simulink library "ITKLib"  (R2022b)
settings: Solver=FixedStepDiscrete  StartTime=0.0  StopTime=10.0  FixedStep=0.01  RelTol=1e-3  EnableMultiTasking=on
values from neighbouring files (symbols this model uses):
  Glb_WhlRollgRd_SC = single(0.36)    [init_Global.m]
undefined symbols (not defined in the file or in its folder): docblock, SlDemoSign, SlDemoSign_Positive_SC, TaskTime_100ms_SC, TaskTime_10ms_SC, VehRefSpd_vMaxRefSpd_C
libraries: simulink x51, $bdroot x45, ITKLib_V14 x1
(part 5 of 10)

== system ITKLib/BasicOperators/SinDeg ==
  deg : Inport
  1-D Lookup Table1 : Lookup_n-D  NumberOfTableDimensions=1  BreakpointsForDimension1=[0,5,10,15,20,25,30,35,40,45,50,55,60,65,70,75,80,85,90]  BreakpointsForDimension1DataTypeStr=single  Table=[0,0.0871557427476582,0.173648177666930,0.258819045102521,0.342020143325669,0.422618261740699,0.500000000000000,0.573576436351046,0.642787609686539,0.707106781186548,0.766044443118978,0.819152044288992,0.866025403784439,0.906307787036650,0.939692620785908,0.965925826289068,0.984807753012208,0.996194698091746,1]  TableDataTypeStr=single  IntermediateResultsDataTypeStr=single  ExtrapMethod=Clip  UseLastTableValue=on  InternalRulePriority=Speed  OutDataTypeStr=single  RndMeth=Simplest  FractionDataTypeStr=single
      settings: AttributesFormatString=|
      | input = %<BreakpointsForDimension1>
      | output = %<Table>
      | extrapolation-use end values: %<UseLastTableValue>
  1-D Lookup Table2 : Lookup_n-D  NumberOfTableDimensions=1  BreakpointsForDimension1=[0,5,10,15,20,25,30,35,40,45,50,55,60,65,70,75,80,85,90]  BreakpointsForDimension1DataTypeStr=single  Table=[0,0.0871557427476582,0.173648177666930,0.258819045102521,0.342020143325669,0.422618261740699,0.500000000000000,0.573576436351046,0.642787609686539,0.707106781186548,0.766044443118978,0.819152044288992,0.866025403784439,0.906307787036650,0.939692620785908,0.965925826289068,0.984807753012208,0.996194698091746,1]  TableDataTypeStr=single  IntermediateResultsDataTypeStr=single  ExtrapMethod=Clip  UseLastTableValue=on  InternalRulePriority=Speed  OutDataTypeStr=single  RndMeth=Simplest  FractionDataTypeStr=single
      settings: AttributesFormatString=|
      | input = %<BreakpointsForDimension1>
      | output = %<Table>
      | extrapolation-use end values: %<UseLastTableValue>
  AbsITK : $bdroot/BasicOperators/AbsITK
  AbsITK1 : $bdroot/BasicOperators/AbsITK
  Divide : Product  Inputs=*/  InputSameDT=on  RndMeth=Zero  SaturateOnIntegerOverflow=on
  GreaterOrEqual{,1..3} (4 alike) : RelationalOperator  OutDataTypeStr=boolean
  GreaterOrEqual4 : RelationalOperator  Operator=<=  OutDataTypeStr=boolean
  GreaterOrEqual5 : RelationalOperator  Operator=<=  OutDataTypeStr=boolean
  GreaterOrEqual6 : RelationalOperator  Operator=<=  OutDataTypeStr=boolean
  Multiport Switch{1..4} (4 alike) : MultiPortSwitch  Inputs=4  SaturateOnIntegerOverflow=off  InputSameDT=off
  Product : Product  InputSameDT=on  RndMeth=Zero  SaturateOnIntegerOverflow=on
  Product1 : Product  InputSameDT=on  RndMeth=Zero  SaturateOnIntegerOverflow=on
  Product2 : Product  InputSameDT=on  RndMeth=Zero  SaturateOnIntegerOverflow=on
  Rounding Function : Rounding  Operator=fix
  Subtract{,1..3} (4 alike) : Sum  Inputs=+-  InputSameDT=on  SaturateOnIntegerOverflow=on
  Subtract4 : Sum  InputSameDT=on  SaturateOnIntegerOverflow=on
  Subtract5 : Sum  InputSameDT=on  SaturateOnIntegerOverflow=on
  Switch{1..7} (7 alike) : Switch  Criteria=u2 ~= 0  SaturateOnIntegerOverflow=off  InputSameDT=off
      settings: AttributesFormatString=Criteria : %<Criteria>
  single1 : Constant  Value=360  OutDataTypeStr=single
      settings: AttributesFormatString=%<OutDataTypeStr>
  single{6,10,14,17} (4 alike) : Constant  Value=180  OutDataTypeStr=single
      settings: AttributesFormatString=%<OutDataTypeStr>
  single11 : Constant  Value=90  OutDataTypeStr=single
      settings: AttributesFormatString=%<OutDataTypeStr>
  single12 : Constant  Value=270  OutDataTypeStr=single
      settings: AttributesFormatString=%<OutDataTypeStr>
  single15 : Constant  Value=360  OutDataTypeStr=single
      settings: AttributesFormatString=%<OutDataTypeStr>
  single19 : Constant  Value=360  OutDataTypeStr=single
      settings: AttributesFormatString=%<OutDataTypeStr>
  single2 : Constant  Value=0  OutDataTypeStr=single
      settings: AttributesFormatString=%<OutDataTypeStr>
  single20 : Constant  OutDataTypeStr=single
      settings: AttributesFormatString=%<OutDataTypeStr>
  single21 : Constant  Value=-1  OutDataTypeStr=single
      settings: AttributesFormatString=%<OutDataTypeStr>
  single3 : Constant  Value=-180  OutDataTypeStr=single
      settings: AttributesFormatString=%<OutDataTypeStr>
  single4 : Constant  Value=-90  OutDataTypeStr=single
      settings: AttributesFormatString=%<OutDataTypeStr>
  single5 : Constant  Value=-270  OutDataTypeStr=single
      settings: AttributesFormatString=%<OutDataTypeStr>
  single7 : Constant  OutDataTypeStr=single
      settings: AttributesFormatString=%<OutDataTypeStr>
  single8 : Constant  Value=-1  OutDataTypeStr=single
      settings: AttributesFormatString=%<OutDataTypeStr>
  uint1 : Constant  OutDataTypeStr=uint8
      settings: AttributesFormatString=%<OutDataTypeStr>
  uint2 : Constant  Value=4  OutDataTypeStr=uint8
      settings: AttributesFormatString=%<OutDataTypeStr>
  uint3 : Constant  Value=3  OutDataTypeStr=uint8
      settings: AttributesFormatString=%<OutDataTypeStr>
  uint4 : Constant  Value=2  OutDataTypeStr=uint8
      settings: AttributesFormatString=%<OutDataTypeStr>
  uint5 : Constant  OutDataTypeStr=uint8
      settings: AttributesFormatString=%<OutDataTypeStr>
  uint6 : Constant  Value=2  OutDataTypeStr=uint8
      settings: AttributesFormatString=%<OutDataTypeStr>
  uint7 : Constant  Value=3  OutDataTypeStr=uint8
      settings: AttributesFormatString=%<OutDataTypeStr>
  uint8 : Constant  Value=4  OutDataTypeStr=uint8
      settings: AttributesFormatString=%<OutDataTypeStr>
  out : Outport
  wires:
  Subtract2/1 -> Multiport Switch1/5
  single15/1 -> Subtract2/1
  Subtract1/1 -> Multiport Switch1/4
  single14/1 -> Subtract1/2
  single8/1 -> Multiport Switch2/4, Multiport Switch2/5
  single7/1 -> Multiport Switch2/2, Multiport Switch2/3
  Product1/1 -> Switch1/1
  Multiport Switch2/1 -> Product1/1
  single6/1 -> Subtract/1
  Subtract/1 -> Multiport Switch1/3
  Multiport Switch1/1 -> 1-D Lookup Table2/1
  uint5/1 -> Switch4/3
  uint4/1 -> Switch4/1
  Switch4/1 -> Switch3/3
  GreaterOrEqual2/1 -> Switch4/2
  single11/1 -> GreaterOrEqual2/2
  uint3/1 -> Switch3/1
  GreaterOrEqual1/1 -> Switch3/2
  single10/1 -> GreaterOrEqual1/2
  single12/1 -> GreaterOrEqual/2
  1-D Lookup Table2/1 -> Product1/2
  Switch2/1 -> Multiport Switch2/1, Multiport Switch1/1
  Switch3/1 -> Switch2/3
  uint2/1 -> Switch2/1
  GreaterOrEqual/1 -> Switch2/2
  Rounding Function/1 -> Product/1
  Product/1 -> Subtract3/2
  Divide/1 -> Rounding Function/1
  deg/1 -> Divide/1, Subtract3/1
  single1/1 -> Product/2, Divide/2
  single2/1 -> GreaterOrEqual3/2
  GreaterOrEqual3/1 -> Switch1/2
  Switch1/1 -> out/1
  GreaterOrEqual4/1 -> Switch5/2
  uint1/1 -> Switch5/1
  Switch6/1 -> Switch5/3
  Switch5/1 -> Multiport Switch4/1, Multiport Switch3/1
  1-D Lookup Table1/1 -> Product2/2
  single5/1 -> GreaterOrEqual4/2
  single3/1 -> GreaterOrEqual5/2
  GreaterOrEqual5/1 -> Switch6/2
  uint6/1 -> Switch6/1
  single4/1 -> GreaterOrEqual6/2
  GreaterOrEqual6/1 -> Switch7/2
  Switch7/1 -> Switch6/3
  uint7/1 -> Switch7/1
  uint8/1 -> Switch7/3
  Multiport Switch3/1 -> 1-D Lookup Table1/1
  Subtract4/1 -> Multiport Switch3/2
  Multiport Switch4/1 -> Product2/1
  Product2/1 -> Switch1/3
  single20/1 -> Multiport Switch4/3, Multiport Switch4/2
  single21/1 -> Multiport Switch4/5, Multiport Switch4/4
  Subtract3/1 -> GreaterOrEqual3/1, AbsITK1/1, Subtract5/1, Subtract4/1, GreaterOrEqual6/1, GreaterOrEqual5/1, GreaterOrEqual4/1, Subtract2/2, Subtract1/1, Subtract/2, Multiport Switch1/2, GreaterOrEqual2/1, GreaterOrEqual1/1, GreaterOrEqual/1
  single19/1 -> Subtract4/2
  single17/1 -> Subtract5/2
  Subtract5/1 -> AbsITK/1, Multiport Switch3/4
  AbsITK/1 -> Multiport Switch3/3
  AbsITK1/1 -> Multiport Switch3/5

== system ITKLib/BasicOperators/SingleToInt ==
  In : Inport  OutDataTypeStr=single
  FL : Inport  Port=2  OutDataTypeStr=single
  DataTypeConversion1 : DataTypeConversion  OutDataTypeStr=int32  RndMeth=Nearest
  Pow1 : Math  Operator=pow  SignedPower=on  RndMeth=Zero
  Product : Product  InputSameDT=on  SaturateOnIntegerOverflow=on
  single1 : Constant  Value=2  OutDataTypeStr=single  SampleTime=-1
      settings: AttributesFormatString=%<OutDataTypeStr>
  Out : Outport  OutDataTypeStr=int32
  wires:
  Product/1 -> DataTypeConversion1/1
  Pow1/1 -> Product/2
  single1/1 -> Pow1/1
  DataTypeConversion1/1 -> Out/1
  In/1 -> Product/1
  FL/1 -> Pow1/2

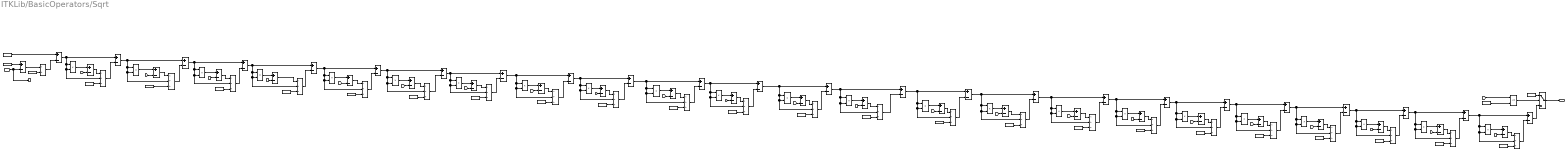
== system ITKLib/BasicOperators/Sqrt ==
  note: 牛顿法的迭代过程：
      | 对于任意方程F(X) = 0, 牛顿法的迭代过程可以描述为
      | Xn+1 = Xn - F(Xn) / F'(Xn)
  In : Inport
  Divide : Product  Inputs=*/  InputSameDT=on  SaturateOnIntegerOverflow=on
  Divide{1..23} (23 alike) : Product  Inputs=*//  InputSameDT=on  SaturateOnIntegerOverflow=on
  GreaterOrEqual : RelationalOperator  Operator=<=  OutDataTypeStr=boolean
  Product{,1..22} (23 alike) : Product  InputSameDT=on  SaturateOnIntegerOverflow=on
  Subtract{,1..47} (48 alike) : Sum  Inputs=+-  InputSameDT=on  SaturateOnIntegerOverflow=on
  Switch : Switch  Criteria=u2 ~= 0  SaturateOnIntegerOverflow=off  InputSameDT=off
      settings: AttributesFormatString=Criteria : %<Criteria>
  single : Constant  Value=0  OutDataTypeStr=single
      settings: AttributesFormatString=%<OutDataTypeStr>
  single1 : Constant  Value=0  OutDataTypeStr=single
      settings: AttributesFormatString=%<OutDataTypeStr>
  single{2,5..27} (24 alike) : Constant  Value=2  OutDataTypeStr=single
      settings: AttributesFormatString=%<OutDataTypeStr>
  single3 : Constant  Value=4  OutDataTypeStr=single
      settings: AttributesFormatString=%<OutDataTypeStr>
  single4 : Constant  Value=4  OutDataTypeStr=single
      settings: AttributesFormatString=%<OutDataTypeStr>
  Sqrt : Outport
  wires:
  single21/1 -> Divide17/3
  Product15/1 -> Subtract33/1
  Subtract36/1 -> Divide17/1
  [In] -> Subtract36/2
  Subtract22/1 -> Subtract24/1, Product11/1, Product11/2, Divide12/2
  Subtract32/1 -> Divide17/2, Product16/2, Product16/1, Subtract35/1
  Subtract28/1 -> Subtract30/1, Divide15/2, Product14/2, Product14/1
  single13/1 -> Divide9/3
  Subtract6/1 -> Divide2/1
  Subtract2/1 -> Subtract5/1, Product1/1, Divide2/2, Product1/2
  Subtract24/1 -> Divide13/2, Product12/2, Product12/1, Subtract26/1
  [In] -> Subtract27/2
  Product13/1 -> Subtract29/1
  single18/1 -> Divide14/3
  Divide17/1 -> Subtract35/2
  Product12/1 -> Subtract27/1
  Subtract8/1 -> Divide3/1
  Divide11/1 -> Subtract22/2
  Product4/1 -> Subtract4/1
  single12/1 -> Divide8/3
  Product1/1 -> Subtract6/1
  Subtract20/1 -> Divide11/2, Product10/2, Product10/1, Subtract22/1
  Subtract25/1 -> Divide12/1
  Subtract23/1 -> Divide11/1
  Divide12/1 -> Subtract24/2
  [In] -> Subtract23/2
  Product8/1 -> Subtract19/1
  [In] -> Subtract17/2
  [In] -> Subtract10/2
  Product6/1 -> Subtract15/1
  Subtract19/1 -> Divide9/1
  single1/1 -> Switch/1
  Subtract21/1 -> Divide10/1
  Subtract11/1 -> Subtract12/1, Product5/1, Divide6/2, Product5/2
  Divide6/1 -> Subtract12/2
  Subtract4/1 -> Divide5/1
  single4/1 -> Divide/2
  Subtract17/1 -> Divide8/1
  Product14/1 -> Subtract31/1
  Divide/1 -> Subtract/2
  Divide3/1 -> Subtract7/2
  single14/1 -> Divide10/3
  GreaterOrEqual/1 -> Switch/2
  [In] -> Subtract13/2
  Product/1 -> Subtract3/1
  single8/1 -> Divide4/3
  Subtract12/1 -> Subtract14/1, Product6/1, Product6/2, Divide7/2
  Divide4/1 -> Subtract9/2
  single5/1 -> Divide1/3
  Divide8/1 -> Subtract16/2
  Divide7/1 -> Subtract14/2
  [In] -> Subtract3/2
  Subtract9/1 -> Divide5/2, Product4/2, Product4/1, Subtract11/1
  single16/1 -> Divide12/3
  Divide1/1 -> Subtract2/2
  [In] -> Subtract45/2
  [In] -> Subtract47/2
  [In] -> Subtract25/2
  Subtract45/1 -> Divide22/1
  single7/1 -> Divide3/3
  Product21/1 -> Subtract45/1
  Divide14/1 -> Subtract28/2
  Subtract44/1 -> Divide23/2, Product22/2, Product22/1, Subtract46/1
  [In] -> Subtract37/2
  single23/1 -> Divide19/3
  Subtract34/1 -> Divide19/2, Product18/2, Product18/1, Subtract38/1
  single27/1 -> Divide23/3
  Subtract1/1 -> Divide/1
  Subtract18/1 -> Subtract20/1, Product9/1, Product9/2, Divide10/2
  [In] -> Subtract29/2
  Subtract/1 -> Subtract2/1, Product/1, Divide1/2, Product/2
  Subtract43/1 -> Divide21/1
  Divide16/1 -> Subtract32/2
  Divide2/1 -> Subtract5/2
  single25/1 -> Divide21/3
  [In] -> Subtract6/2
  [In] -> Subtract31/2
  Subtract41/1 -> Divide20/1
  Subtract14/1 -> Subtract16/1, Product7/1, Product7/2, Divide8/2
  Switch/1 -> Sqrt/1
  Subtract16/1 -> Product8/2, Divide9/2, Product8/1, Subtract18/1
  Product22/1 -> Subtract47/1
  single26/1 -> Divide22/3
  Subtract42/1 -> Subtract44/1, Product21/1, Product21/2, Divide22/2
  single15/1 -> Divide11/3
  [In] -> Subtract43/2
  Divide23/1 -> Subtract46/2
  Divide22/1 -> Subtract44/2
  single9/1 -> Divide5/3
  Subtract3/1 -> Divide1/1
  [In] -> Subtract33/2
  single3/1 -> Subtract1/1
  Product20/1 -> Subtract43/1
  single20/1 -> Divide16/3
  Subtract10/1 -> Divide4/1
  [In] -> Subtract21/2
  Divide20/1 -> Subtract40/2
  Product18/1 -> Subtract39/1
  single2/1 -> Subtract/1
  single6/1 -> Divide2/3
  Subtract40/1 -> Divide21/2, Product20/2, Product20/1, Subtract42/1
  Product2/1 -> Subtract8/1
  In/1 -> [In], Subtract1/2
  Divide10/1 -> Subtract20/2
  Divide21/1 -> Subtract42/2
  Product10/1 -> Subtract23/1
  Subtract13/1 -> Divide6/1
  Product19/1 -> Subtract41/1
  [In] -> Subtract41/2
  Subtract30/1 -> Product15/1, Product15/2, Divide16/2, Subtract32/1
  [In] -> Subtract15/2
  Subtract38/1 -> Subtract40/1, Product19/1, Product19/2, Divide20/2
  Subtract5/1 -> Divide3/2, Product2/2, Product2/1, Subtract7/1
  Divide9/1 -> Subtract18/2
  [In] -> Subtract19/2
  Subtract39/1 -> Divide19/1
  single/1 -> GreaterOrEqual/2
  single22/1 -> Divide18/3
  Product9/1 -> Subtract21/1
  [In] -> GreaterOrEqual/1
  Product3/1 -> Subtract10/1
  Subtract29/1 -> Divide14/1
  Product5/1 -> Subtract13/1
  Subtract33/1 -> Divide16/1
  single24/1 -> Divide20/3
  Subtract46/1 -> Switch/3
  [In] -> Subtract8/2
  Subtract26/1 -> Product13/1, Product13/2, Divide14/2, Subtract28/1
  Product11/1 -> Subtract25/1
  Product16/1 -> Subtract36/1
  Subtract27/1 -> Divide13/1
  single19/1 -> Divide15/3
  Subtract35/1 -> Subtract34/1, Product17/1, Product17/2, Divide18/2
  single17/1 -> Divide13/3
  Divide18/1 -> Subtract34/2
  [In] -> Subtract4/2
  Subtract31/1 -> Divide15/1
  single10/1 -> Divide6/3
  [In] -> Subtract39/2
  Subtract47/1 -> Divide23/1
  Divide5/1 -> Subtract11/2
  Subtract7/1 -> Subtract9/1, Product3/1, Divide4/2, Product3/2
  Product17/1 -> Subtract37/1
  Subtract37/1 -> Divide18/1
  Product7/1 -> Subtract17/1
  single11/1 -> Divide7/3
  Subtract15/1 -> Divide7/1
  Divide15/1 -> Subtract30/2
  Divide19/1 -> Subtract38/2
  Divide13/1 -> Subtract26/2

== system ITKLib/BasicOperators/TanDeg ==
  deg : Inport
  1-D Lookup Table2 : Lookup_n-D  NumberOfTableDimensions=1  BreakpointsForDimension1=[0,5,10,15,20,25,30,35,40,45,50,55,60,65,70,75,80,85,86,87,88,89,89.5,89.9]  BreakpointsForDimension1DataTypeStr=single  Table=[0,0.0874886635259240,0.176326980708465,0.267949192431123,0.363970234266202,0.466307658154999,0.577350269189626,0.700207538209710,0.839099631177280,1.00000000000000,1.19175359259421,1.42814800674211,1.73205080756888,2.14450692050956,2.74747741945462,3.73205080756888,5.67128181961771,11.4300523027613,14.3007,19.0811,28.6363,57.29,114.5887,573]  TableDataTypeStr=single  IntermediateResultsDataTypeStr=single  ExtrapMethod=Clip  UseLastTableValue=on  InternalRulePriority=Speed  OutDataTypeStr=single  RndMeth=Simplest  FractionDataTypeStr=single
      settings: AttributesFormatString=|
      | input = %<BreakpointsForDimension1>
      | output = %<Table>
      | extrapolation-use end values: %<UseLastTableValue>
  1-D Lookup Table3 : Lookup_n-D  NumberOfTableDimensions=1  BreakpointsForDimension1=[0,5,10,15,20,25,30,35,40,45,50,55,60,65,70,75,80,85,86,87,88,89,89.5,89.9]  BreakpointsForDimension1DataTypeStr=single  Table=[0,0.0874886635259240,0.176326980708465,0.267949192431123,0.363970234266202,0.466307658154999,0.577350269189626,0.700207538209710,0.839099631177280,1.00000000000000,1.19175359259421,1.42814800674211,1.73205080756888,2.14450692050956,2.74747741945462,3.73205080756888,5.67128181961771,11.4300523027613,14.3007,19.0811,28.6363,57.29,114.5887,573]  TableDataTypeStr=single  IntermediateResultsDataTypeStr=single  ExtrapMethod=Clip  UseLastTableValue=on  InternalRulePriority=Speed  OutDataTypeStr=single  RndMeth=Simplest  FractionDataTypeStr=single
      settings: AttributesFormatString=|
      | input = %<BreakpointsForDimension1>
      | output = %<Table>
      | extrapolation-use end values: %<UseLastTableValue>
  AbsITK : $bdroot/BasicOperators/AbsITK
  AbsITK1 : $bdroot/BasicOperators/AbsITK
  Divide : Product  Inputs=*/  InputSameDT=on  RndMeth=Zero  SaturateOnIntegerOverflow=on
  GreaterOrEqual{,1..2,6} (4 alike) : RelationalOperator  OutDataTypeStr=boolean
  GreaterOrEqual7 : RelationalOperator  Operator=<=  OutDataTypeStr=boolean
  GreaterOrEqual8 : RelationalOperator  Operator=<=  OutDataTypeStr=boolean
  GreaterOrEqual9 : RelationalOperator  Operator=<=  OutDataTypeStr=boolean
  Multiport Switch{1..2,5..6} (4 alike) : MultiPortSwitch  Inputs=4  SaturateOnIntegerOverflow=off  InputSameDT=off
  Product : Product  InputSameDT=on  RndMeth=Zero  SaturateOnIntegerOverflow=on
  Product1 : Product  InputSameDT=on  RndMeth=Zero  SaturateOnIntegerOverflow=on
  Product3 : Product  InputSameDT=on  RndMeth=Zero  SaturateOnIntegerOverflow=on
  Rounding Function : Rounding  Operator=fix
  Subtract{,1..2,6} (4 alike) : Sum  Inputs=+-  InputSameDT=on  SaturateOnIntegerOverflow=on
  Subtract7 : Sum  InputSameDT=on  SaturateOnIntegerOverflow=on
  Subtract8 : Sum  InputSameDT=on  SaturateOnIntegerOverflow=on
  Switch{1..4,8..10} (7 alike) : Switch  Criteria=u2 ~= 0  SaturateOnIntegerOverflow=off  InputSameDT=off
      settings: AttributesFormatString=Criteria : %<Criteria>
  single{1,5,8,25} (4 alike) : Constant  Value=-1  OutDataTypeStr=single
      settings: AttributesFormatString=%<OutDataTypeStr>
  single{6,10,14,21} (4 alike) : Constant  Value=180  OutDataTypeStr=single
      settings: AttributesFormatString=%<OutDataTypeStr>
  single11 : Constant  Value=90  OutDataTypeStr=single
      settings: AttributesFormatString=%<OutDataTypeStr>
  single12 : Constant  Value=270  OutDataTypeStr=single
      settings: AttributesFormatString=%<OutDataTypeStr>
  single15 : Constant  Value=360  OutDataTypeStr=single
      settings: AttributesFormatString=%<OutDataTypeStr>
  single{2,4,7,24} (4 alike) : Constant  OutDataTypeStr=single
      settings: AttributesFormatString=%<OutDataTypeStr>
  single22 : Constant  Value=360  OutDataTypeStr=single
      settings: AttributesFormatString=%<OutDataTypeStr>
  single23 : Constant  Value=0  OutDataTypeStr=single
      settings: AttributesFormatString=%<OutDataTypeStr>
  single27 : Constant  Value=-180  OutDataTypeStr=single
      settings: AttributesFormatString=%<OutDataTypeStr>
  single28 : Constant  Value=-90  OutDataTypeStr=single
      settings: AttributesFormatString=%<OutDataTypeStr>
  single29 : Constant  Value=-270  OutDataTypeStr=single
      settings: AttributesFormatString=%<OutDataTypeStr>
  single3 : Constant  Value=360  OutDataTypeStr=single
      settings: AttributesFormatString=%<OutDataTypeStr>
  uint1 : Constant  OutDataTypeStr=uint8
      settings: AttributesFormatString=%<OutDataTypeStr>
  uint10 : Constant  Value=2  OutDataTypeStr=uint8
      settings: AttributesFormatString=%<OutDataTypeStr>
  uint11 : Constant  Value=3  OutDataTypeStr=uint8
      settings: AttributesFormatString=%<OutDataTypeStr>
  uint12 : Constant  Value=4  OutDataTypeStr=uint8
      settings: AttributesFormatString=%<OutDataTypeStr>
  uint2 : Constant  Value=4  OutDataTypeStr=uint8
      settings: AttributesFormatString=%<OutDataTypeStr>
  uint3 : Constant  Value=3  OutDataTypeStr=uint8
      settings: AttributesFormatString=%<OutDataTypeStr>
  uint4 : Constant  Value=2  OutDataTypeStr=uint8
      settings: AttributesFormatString=%<OutDataTypeStr>
  uint5 : Constant  OutDataTypeStr=uint8
      settings: AttributesFormatString=%<OutDataTypeStr>
  out : Outport
  wires:
  Subtract2/1 -> Multiport Switch1/5
  single15/1 -> Subtract2/1
  Subtract1/1 -> Multiport Switch1/4
  single14/1 -> Subtract1/2
  single8/1 -> Multiport Switch2/5
  single7/1 -> Multiport Switch2/2
  Multiport Switch2/1 -> Product1/1
  single6/1 -> Subtract/1
  Subtract/1 -> Multiport Switch1/3
  Multiport Switch1/1 -> 1-D Lookup Table2/1
  uint5/1 -> Switch4/3
  uint4/1 -> Switch4/1
  Switch4/1 -> Switch3/3
  GreaterOrEqual2/1 -> Switch4/2
  single11/1 -> GreaterOrEqual2/2
  uint3/1 -> Switch3/1
  GreaterOrEqual1/1 -> Switch3/2
  single10/1 -> GreaterOrEqual1/2
  single12/1 -> GreaterOrEqual/2
  1-D Lookup Table2/1 -> Product1/2
  Switch2/1 -> Multiport Switch1/1, Multiport Switch2/1
  Switch3/1 -> Switch2/3
  uint2/1 -> Switch2/1
  GreaterOrEqual/1 -> Switch2/2
  single1/1 -> Multiport Switch2/3
  single2/1 -> Multiport Switch2/4
  single5/1 -> Multiport Switch6/5
  uint11/1 -> Switch10/1
  single24/1 -> Multiport Switch6/2
  single23/1 -> GreaterOrEqual6/2
  deg/1 -> Divide/1, Subtract6/1
  1-D Lookup Table3/1 -> Product3/2
  Multiport Switch5/1 -> 1-D Lookup Table3/1
  Switch8/1 -> Multiport Switch5/1, Multiport Switch6/1
  Product3/1 -> Switch1/3
  single22/1 -> Subtract7/2
  single27/1 -> GreaterOrEqual8/2
  Subtract6/1 -> GreaterOrEqual6/1, AbsITK1/1, Subtract8/1, Subtract7/1, GreaterOrEqual9/1, GreaterOrEqual8/1, GreaterOrEqual7/1, Subtract2/2, Subtract1/1, Subtract/2, Multiport Switch1/2, GreaterOrEqual2/1, GreaterOrEqual1/1, GreaterOrEqual/1
  single21/1 -> Subtract8/2
  GreaterOrEqual7/1 -> Switch8/2
  single25/1 -> Multiport Switch6/3
  Subtract8/1 -> AbsITK/1, Multiport Switch5/4
  uint1/1 -> Switch8/1
  GreaterOrEqual9/1 -> Switch10/2
  Rounding Function/1 -> Product/1
  Multiport Switch6/1 -> Product3/1
  single28/1 -> GreaterOrEqual9/2
  Divide/1 -> Rounding Function/1
  Product/1 -> Subtract6/2
  Subtract7/1 -> Multiport Switch5/2
  Switch9/1 -> Switch8/3
  single3/1 -> Product/2, Divide/2
  GreaterOrEqual8/1 -> Switch9/2
  uint10/1 -> Switch9/1
  uint12/1 -> Switch10/3
  Switch1/1 -> out/1
  Switch10/1 -> Switch9/3
  GreaterOrEqual6/1 -> Switch1/2
  single29/1 -> GreaterOrEqual7/2
  Product1/1 -> Switch1/1
  single4/1 -> Multiport Switch6/4
  AbsITK/1 -> Multiport Switch5/3
  AbsITK1/1 -> Multiport Switch5/5

== system ITKLib/BasicOperators/arccos ==
  u : Inport
  1-D Lookup Table1 : Lookup_n-D  NumberOfTableDimensions=1  BreakpointsForDimension1=[0,0.05,0.1,0.15,0.2,0.25,0.3,0.35,0.4,0.45,0.5,0.55,0.6,0.65,0.7,0.75,0.8,0.85,0.9,0.95,1]  BreakpointsForDimension1DataTypeStr=single  Table=[90,87.1340160174012,84.2608295227332,81.3730734413214,78.4630409671845,75.5224878140701,72.5423968762779,69.5126848852773,66.4218215217982,63.2563160495970,60.0000000000000,56.6329870307682,53.1301023541560,49.4583981264955,45.5729959991943,41.4096221092709,36.8698976458440,31.7883306170516,25.8419327631671,18.1948723387668,0]  TableDataTypeStr=single  IntermediateResultsDataTypeStr=single  ExtrapMethod=Clip  UseLastTableValue=on  InternalRulePriority=Speed  OutDataTypeStr=single  RndMeth=Simplest  FractionDataTypeStr=single
      settings: AttributesFormatString=|
      | input = %<BreakpointsForDimension1>
      | output = %<Table>
      | extrapolation-use end values: %<UseLastTableValue>
  AbsITK : $bdroot/BasicOperators/AbsITK
  Divide1 : Product  Inputs=*/  InputSameDT=on  RndMeth=Zero  SaturateOnIntegerOverflow=on
  GreaterOrEqual3 : RelationalOperator  OutDataTypeStr=boolean
  Product4 : Product  InputSameDT=on  RndMeth=Zero  SaturateOnIntegerOverflow=on
  Subtract : Sum  Inputs=+-  InputSameDT=on  SaturateOnIntegerOverflow=on
  Switch1 : Switch  Criteria=u2 ~= 0  SaturateOnIntegerOverflow=off  InputSameDT=off
      settings: AttributesFormatString=Criteria : %<Criteria>
  single1 : Constant  Value=0  OutDataTypeStr=single
      settings: AttributesFormatString=%<OutDataTypeStr>
  single2 : Constant  Value=180  OutDataTypeStr=single
      settings: AttributesFormatString=%<OutDataTypeStr>
  single3 : Constant  Value=180  OutDataTypeStr=single
      settings: AttributesFormatString=%<OutDataTypeStr>
  single4 : Constant  Value=3.141593  OutDataTypeStr=single
      settings: AttributesFormatString=%<OutDataTypeStr>
  rad : Outport
  wires:
  Switch1/1 -> Divide1/1  "deg"
  GreaterOrEqual3/1 -> Switch1/2
  single2/1 -> Subtract/1
  1-D Lookup Table1/1 -> Subtract/2, Switch1/1
  Subtract/1 -> Switch1/3
  single1/1 -> GreaterOrEqual3/2
  u/1 -> AbsITK/1, GreaterOrEqual3/1
  Divide1/1 -> Product4/1
  single3/1 -> Divide1/2
  single4/1 -> Product4/2
  Product4/1 -> rad/1  "rad"
  AbsITK/1 -> 1-D Lookup Table1/1

== system ITKLib/BasicOperators/arcsin ==
  u : Inport
  1-D Lookup Table1 : Lookup_n-D  NumberOfTableDimensions=1  BreakpointsForDimension1=[0.0000 0.1045 0.2079 0.4067 0.5000 0.5878 0.6691 0.7431 0.8090 0.8660 0.9135 0.9511 0.9781 0.9945 1.0000]  BreakpointsForDimension1DataTypeStr=single  Table=[0.0000 0.1047 0.2094 0.4189 0.5236 0.6283 0.7330 0.8378 0.9425 1.0472 1.1519 1.2566 1.3614 1.4661 1.5708]  TableDataTypeStr=single  IntermediateResultsDataTypeStr=single  ExtrapMethod=Clip  UseLastTableValue=on  InternalRulePriority=Speed  OutDataTypeStr=single  RndMeth=Simplest  FractionDataTypeStr=single
      settings: AttributesFormatString=|
      | input = %<BreakpointsForDimension1>
      | output = %<Table>
      | extrapolation-use end values: %<UseLastTableValue>
  AbsITK : $bdroot/BasicOperators/AbsITK
  GreaterOrEqual3 : RelationalOperator  OutDataTypeStr=boolean
  Product : Product  InputSameDT=on  RndMeth=Zero  SaturateOnIntegerOverflow=on
  Switch1 : Switch  Criteria=u2 ~= 0  SaturateOnIntegerOverflow=off  InputSameDT=off
      settings: AttributesFormatString=Criteria : %<Criteria>
  single1 : Constant  Value=0  OutDataTypeStr=single
      settings: AttributesFormatString=%<OutDataTypeStr>
  single2 : Constant  Value=-1  OutDataTypeStr=single
      settings: AttributesFormatString=%<OutDataTypeStr>
  rad : Outport
  wires:
  single2/1 -> Product/2
  Switch1/1 -> rad/1
  single1/1 -> GreaterOrEqual3/2
  GreaterOrEqual3/1 -> Switch1/2
  u/1 -> AbsITK/1, GreaterOrEqual3/1
  Product/1 -> Switch1/3
  1-D Lookup Table1/1 -> Switch1/1, Product/1
  AbsITK/1 -> 1-D Lookup Table1/1

== system ITKLib/BasicOperators/arctan ==
  u : Inport
  1-D Lookup Table1 : Lookup_n-D  NumberOfTableDimensions=1  BreakpointsForDimension1=[0.0000 0.1051 0.2126 0.4452 0.5774 0.7265 0.9004 1.1106 1.3764 1.7321 2.2461 3.0777 4.7047 9.5147 100.0000]  BreakpointsForDimension1DataTypeStr=single  Table=[0.0000 0.1047 0.2094 0.4189 0.5236 0.6283 0.7330 0.8378 0.9425 1.0472 1.1519 1.2566 1.3614 1.4661 1.5708]  TableDataTypeStr=single  IntermediateResultsDataTypeStr=single  ExtrapMethod=Clip  UseLastTableValue=on  InternalRulePriority=Speed  OutDataTypeStr=single  RndMeth=Simplest  FractionDataTypeStr=single
      settings: AttributesFormatString=|
      | input = %<BreakpointsForDimension1>
      | output = %<Table>
      | extrapolation-use end values: %<UseLastTableValue>
  AbsITK : $bdroot/BasicOperators/AbsITK
  GreaterOrEqual3 : RelationalOperator  OutDataTypeStr=boolean
  Product : Product  InputSameDT=on  RndMeth=Zero  SaturateOnIntegerOverflow=on
  Switch1 : Switch  Criteria=u2 ~= 0  SaturateOnIntegerOverflow=off  InputSameDT=off
      settings: AttributesFormatString=Criteria : %<Criteria>
  single1 : Constant  Value=0  OutDataTypeStr=single
      settings: AttributesFormatString=%<OutDataTypeStr>
  single2 : Constant  Value=-1  OutDataTypeStr=single
      settings: AttributesFormatString=%<OutDataTypeStr>
  rad : Outport
  wires:
  Switch1/1 -> rad/1
  GreaterOrEqual3/1 -> Switch1/2
  1-D Lookup Table1/1 -> Product/1, Switch1/1
  Product/1 -> Switch1/3
  u/1 -> AbsITK/1, GreaterOrEqual3/1
  single1/1 -> GreaterOrEqual3/2
  single2/1 -> Product/2
  AbsITK/1 -> 1-D Lookup Table1/1

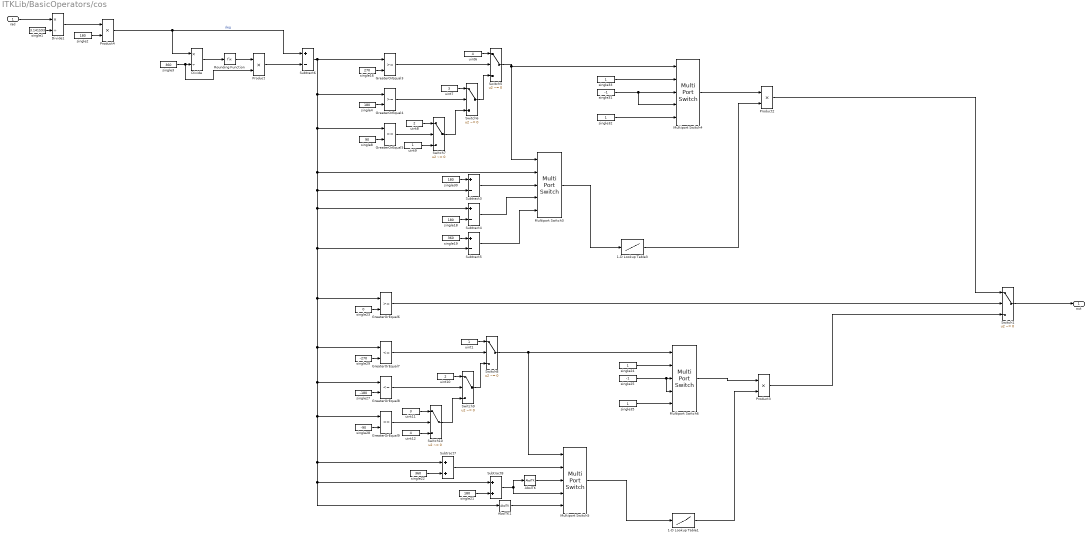
== system ITKLib/BasicOperators/cos ==
  rad : Inport
  1-D Lookup Table1 : Lookup_n-D  NumberOfTableDimensions=1  BreakpointsForDimension1=[0,5,10,15,20,25,30,35,40,45,50,55,60,65,70,75,80,85,90]  BreakpointsForDimension1DataTypeStr=single  Table=[1,0.996194698091746,0.984807753012208,0.965925826289068,0.939692620785908,0.906307787036650,0.866025403784439,0.819152044288992,0.766044443118978,0.707106781186548,0.642787609686539,0.573576436351046,0.500000000000000,0.422618261740699,0.342020143325669,0.258819045102521,0.173648177666930,0.0871557427476584,6.12323399573677e-17]  TableDataTypeStr=single  IntermediateResultsDataTypeStr=single  ExtrapMethod=Clip  UseLastTableValue=on  InternalRulePriority=Speed  OutDataTypeStr=single  RndMeth=Simplest  FractionDataTypeStr=single
      settings: AttributesFormatString=|
      | input = %<BreakpointsForDimension1>
      | output = %<Table>
      | extrapolation-use end values: %<UseLastTableValue>
  1-D Lookup Table3 : Lookup_n-D  NumberOfTableDimensions=1  BreakpointsForDimension1=[0,5,10,15,20,25,30,35,40,45,50,55,60,65,70,75,80,85,90]  BreakpointsForDimension1DataTypeStr=single  Table=[1,0.996194698091746,0.984807753012208,0.965925826289068,0.939692620785908,0.906307787036650,0.866025403784439,0.819152044288992,0.766044443118978,0.707106781186548,0.642787609686539,0.573576436351046,0.500000000000000,0.422618261740699,0.342020143325669,0.258819045102521,0.173648177666930,0.0871557427476584,6.12323399573677e-17]  TableDataTypeStr=single  IntermediateResultsDataTypeStr=single  ExtrapMethod=Clip  UseLastTableValue=on  InternalRulePriority=Speed  OutDataTypeStr=single  RndMeth=Simplest  FractionDataTypeStr=single
      settings: AttributesFormatString=|
      | input = %<BreakpointsForDimension1>
      | output = %<Table>
      | extrapolation-use end values: %<UseLastTableValue>
  AbsITK : $bdroot/BasicOperators/AbsITK
  AbsITK1 : $bdroot/BasicOperators/AbsITK
  Divide : Product  Inputs=*/  InputSameDT=on  RndMeth=Zero  SaturateOnIntegerOverflow=on
  Divide1 : Product  Inputs=*/  InputSameDT=on  RndMeth=Zero  SaturateOnIntegerOverflow=on
  GreaterOrEqual{3..6} (4 alike) : RelationalOperator  OutDataTypeStr=boolean
  GreaterOrEqual7 : RelationalOperator  Operator=<=  OutDataTypeStr=boolean
  GreaterOrEqual8 : RelationalOperator  Operator=<=  OutDataTypeStr=boolean
  GreaterOrEqual9 : RelationalOperator  Operator=<=  OutDataTypeStr=boolean
  Multiport Switch{3..6} (4 alike) : MultiPortSwitch  Inputs=4  SaturateOnIntegerOverflow=off  InputSameDT=off
  Product{,2..4} (4 alike) : Product  InputSameDT=on  RndMeth=Zero  SaturateOnIntegerOverflow=on
  Rounding Function : Rounding  Operator=fix
  Subtract{3..6} (4 alike) : Sum  Inputs=+-  InputSameDT=on  SaturateOnIntegerOverflow=on
  Subtract7 : Sum  InputSameDT=on  SaturateOnIntegerOverflow=on
  Subtract8 : Sum  InputSameDT=on  SaturateOnIntegerOverflow=on
  Switch{1,5..10} (7 alike) : Switch  Criteria=u2 ~= 0  SaturateOnIntegerOverflow=off  InputSameDT=off
      settings: AttributesFormatString=Criteria : %<Criteria>
  single1 : Constant  Value=3.141593  OutDataTypeStr=single
      settings: AttributesFormatString=%<OutDataTypeStr>
  single16 : Constant  Value=270  OutDataTypeStr=single
      settings: AttributesFormatString=%<OutDataTypeStr>
  single{2,4,18,21,30} (5 alike) : Constant  Value=180  OutDataTypeStr=single
      settings: AttributesFormatString=%<OutDataTypeStr>
  single19 : Constant  Value=360  OutDataTypeStr=single
      settings: AttributesFormatString=%<OutDataTypeStr>
  single22 : Constant  Value=360  OutDataTypeStr=single
      settings: AttributesFormatString=%<OutDataTypeStr>
  single23 : Constant  Value=0  OutDataTypeStr=single
      settings: AttributesFormatString=%<OutDataTypeStr>
  single{24,32..33,35} (4 alike) : Constant  OutDataTypeStr=single
      settings: AttributesFormatString=%<OutDataTypeStr>
  single25 : Constant  Value=-1  OutDataTypeStr=single
      settings: AttributesFormatString=%<OutDataTypeStr>
  single27 : Constant  Value=-180  OutDataTypeStr=single
      settings: AttributesFormatString=%<OutDataTypeStr>
  single28 : Constant  Value=-90  OutDataTypeStr=single
      settings: AttributesFormatString=%<OutDataTypeStr>
  single29 : Constant  Value=-270  OutDataTypeStr=single
      settings: AttributesFormatString=%<OutDataTypeStr>
  single3 : Constant  Value=360  OutDataTypeStr=single
      settings: AttributesFormatString=%<OutDataTypeStr>
  single31 : Constant  Value=-1  OutDataTypeStr=single
      settings: AttributesFormatString=%<OutDataTypeStr>
  single8 : Constant  Value=90  OutDataTypeStr=single
      settings: AttributesFormatString=%<OutDataTypeStr>
  uint1 : Constant  OutDataTypeStr=uint8
      settings: AttributesFormatString=%<OutDataTypeStr>
  uint10 : Constant  Value=2  OutDataTypeStr=uint8
      settings: AttributesFormatString=%<OutDataTypeStr>
  uint11 : Constant  Value=3  OutDataTypeStr=uint8
      settings: AttributesFormatString=%<OutDataTypeStr>
  uint12 : Constant  Value=4  OutDataTypeStr=uint8
      settings: AttributesFormatString=%<OutDataTypeStr>
  uint6 : Constant  Value=4  OutDataTypeStr=uint8
      settings: AttributesFormatString=%<OutDataTypeStr>
  uint7 : Constant  Value=3  OutDataTypeStr=uint8
      settings: AttributesFormatString=%<OutDataTypeStr>
  uint8 : Constant  Value=2  OutDataTypeStr=uint8
      settings: AttributesFormatString=%<OutDataTypeStr>
  uint9 : Constant  OutDataTypeStr=uint8
      settings: AttributesFormatString=%<OutDataTypeStr>
  out : Outport
  wires:
  GreaterOrEqual4/1 -> Switch6/2
  Switch7/1 -> Switch6/3
  uint1/1 -> Switch8/1
  single27/1 -> GreaterOrEqual8/2
  GreaterOrEqual6/1 -> Switch1/2
  1-D Lookup Table3/1 -> Product2/2
  single21/1 -> Subtract8/2
  single18/1 -> Subtract4/2
  Multiport Switch4/1 -> Product2/1
  AbsITK/1 -> Multiport Switch5/3
  single3/1 -> Product/2, Divide/2
  uint9/1 -> Switch7/3
  1-D Lookup Table1/1 -> Product3/2
  Multiport Switch5/1 -> 1-D Lookup Table1/1
  Multiport Switch3/1 -> 1-D Lookup Table3/1
  single29/1 -> GreaterOrEqual7/2
  Rounding Function/1 -> Product/1
  GreaterOrEqual3/1 -> Switch5/2
  Multiport Switch6/1 -> Product3/1
  Switch6/1 -> Switch5/3
  single30/1 -> Subtract3/1
  GreaterOrEqual8/1 -> Switch9/2
  Subtract8/1 -> AbsITK/1, Multiport Switch5/4
  uint7/1 -> Switch6/1
  uint10/1 -> Switch9/1
  Product/1 -> Subtract6/2
  single4/1 -> GreaterOrEqual4/2
  Switch5/1 -> Multiport Switch4/1, Multiport Switch3/1
  single16/1 -> GreaterOrEqual3/2
  Switch9/1 -> Switch8/3
  Product3/1 -> Switch1/3
  Product2/1 -> Switch1/1
  uint12/1 -> Switch10/3
  Switch8/1 -> Multiport Switch5/1, Multiport Switch6/1
  Product4/1 -> Divide/1, Subtract6/1  "deg"
  Subtract5/1 -> Multiport Switch3/5
  single23/1 -> GreaterOrEqual6/2
  single35/1 -> Multiport Switch6/5
  GreaterOrEqual5/1 -> Switch7/2
  Divide/1 -> Rounding Function/1
  Subtract4/1 -> Multiport Switch3/4
  uint6/1 -> Switch5/1
  uint11/1 -> Switch10/1
  GreaterOrEqual9/1 -> Switch10/2
  single24/1 -> Multiport Switch6/2
  single19/1 -> Subtract5/1
  single31/1 -> Multiport Switch4/3, Multiport Switch4/4
  Subtract3/1 -> Multiport Switch3/3
  single32/1 -> Multiport Switch4/5
  Switch10/1 -> Switch9/3
  GreaterOrEqual7/1 -> Switch8/2
  Subtract7/1 -> Multiport Switch5/2
  single22/1 -> Subtract7/2
  single28/1 -> GreaterOrEqual9/2
  Switch1/1 -> out/1
  single33/1 -> Multiport Switch4/2
  single8/1 -> GreaterOrEqual5/2
  Subtract6/1 -> GreaterOrEqual6/1, AbsITK1/1, Subtract8/1, Subtract7/1, GreaterOrEqual9/1, GreaterOrEqual8/1, GreaterOrEqual7/1, Subtract5/2, Subtract4/1, Subtract3/2, Multiport Switch3/2, GreaterOrEqual5/1, GreaterOrEqual4/1, GreaterOrEqual3/1
  single25/1 -> Multiport Switch6/3, Multiport Switch6/4
  uint8/1 -> Switch7/1
  Divide1/1 -> Product4/1
  single1/1 -> Divide1/2
  single2/1 -> Product4/2
  rad/1 -> Divide1/1
  AbsITK1/1 -> Multiport Switch5/5

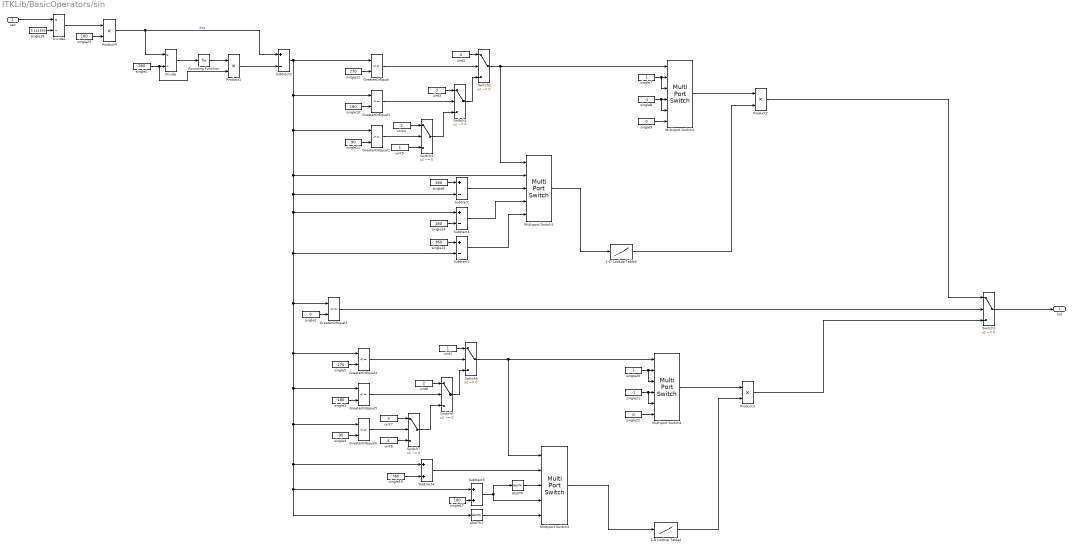
== system ITKLib/BasicOperators/sin ==
  rad : Inport
  1-D Lookup Table2 : Lookup_n-D  NumberOfTableDimensions=1  BreakpointsForDimension1=[0,5,10,15,20,25,30,35,40,45,50,55,60,65,70,75,80,85,90]  BreakpointsForDimension1DataTypeStr=single  Table=[0,0.0871557427476582,0.173648177666930,0.258819045102521,0.342020143325669,0.422618261740699,0.500000000000000,0.573576436351046,0.642787609686539,0.707106781186548,0.766044443118978,0.819152044288992,0.866025403784439,0.906307787036650,0.939692620785908,0.965925826289068,0.984807753012208,0.996194698091746,1]  TableDataTypeStr=single  IntermediateResultsDataTypeStr=single  ExtrapMethod=Clip  UseLastTableValue=on  InternalRulePriority=Speed  OutDataTypeStr=single  RndMeth=Simplest  FractionDataTypeStr=single
      settings: AttributesFormatString=|
      | input = %<BreakpointsForDimension1>
      | output = %<Table>
      | extrapolation-use end values: %<UseLastTableValue>
  1-D Lookup Table3 : Lookup_n-D  NumberOfTableDimensions=1  BreakpointsForDimension1=[0,5,10,15,20,25,30,35,40,45,50,55,60,65,70,75,80,85,90]  BreakpointsForDimension1DataTypeStr=single  Table=[0,0.0871557427476582,0.173648177666930,0.258819045102521,0.342020143325669,0.422618261740699,0.500000000000000,0.573576436351046,0.642787609686539,0.707106781186548,0.766044443118978,0.819152044288992,0.866025403784439,0.906307787036650,0.939692620785908,0.965925826289068,0.984807753012208,0.996194698091746,1]  TableDataTypeStr=single  IntermediateResultsDataTypeStr=single  ExtrapMethod=Clip  UseLastTableValue=on  InternalRulePriority=Speed  OutDataTypeStr=single  RndMeth=Simplest  FractionDataTypeStr=single
      settings: AttributesFormatString=|
      | input = %<BreakpointsForDimension1>
      | output = %<Table>
      | extrapolation-use end values: %<UseLastTableValue>
  AbsITK : $bdroot/BasicOperators/AbsITK
  AbsITK1 : $bdroot/BasicOperators/AbsITK
  Divide : Product  Inputs=*/  InputSameDT=on  RndMeth=Zero  SaturateOnIntegerOverflow=on
  Divide1 : Product  Inputs=*/  InputSameDT=on  RndMeth=Zero  SaturateOnIntegerOverflow=on
  GreaterOrEqual{,1..3} (4 alike) : RelationalOperator  OutDataTypeStr=boolean
  GreaterOrEqual4 : RelationalOperator  Operator=<=  OutDataTypeStr=boolean
  GreaterOrEqual5 : RelationalOperator  Operator=<=  OutDataTypeStr=boolean
  GreaterOrEqual6 : RelationalOperator  Operator=<=  OutDataTypeStr=boolean
  Multiport Switch1 : MultiPortSwitch  Inputs=4  SaturateOnIntegerOverflow=off  InputSameDT=off
  Multiport Switch2 : MultiPortSwitch  Inputs=5  SaturateOnIntegerOverflow=off  InputSameDT=off
  Multiport Switch3 : MultiPortSwitch  Inputs=4  SaturateOnIntegerOverflow=off  InputSameDT=off
  Multiport Switch4 : MultiPortSwitch  Inputs=5  SaturateOnIntegerOverflow=off  InputSameDT=off
  Product{1..4} (4 alike) : Product  InputSameDT=on  RndMeth=Zero  SaturateOnIntegerOverflow=on
  Rounding Function : Rounding  Operator=fix
  Subtract{,1..3} (4 alike) : Sum  Inputs=+-  InputSameDT=on  SaturateOnIntegerOverflow=on
  Subtract4 : Sum  InputSameDT=on  SaturateOnIntegerOverflow=on
  Subtract5 : Sum  InputSameDT=on  SaturateOnIntegerOverflow=on
  Switch{1..7} (7 alike) : Switch  Criteria=u2 ~= 0  SaturateOnIntegerOverflow=off  InputSameDT=off
      settings: AttributesFormatString=Criteria : %<Criteria>
  single1 : Constant  Value=360  OutDataTypeStr=single
      settings: AttributesFormatString=%<OutDataTypeStr>
  single{6,10,14,17,23} (5 alike) : Constant  Value=180  OutDataTypeStr=single
      settings: AttributesFormatString=%<OutDataTypeStr>
  single11 : Constant  Value=90  OutDataTypeStr=single
      settings: AttributesFormatString=%<OutDataTypeStr>
  single12 : Constant  Value=270  OutDataTypeStr=single
      settings: AttributesFormatString=%<OutDataTypeStr>
  single15 : Constant  Value=360  OutDataTypeStr=single
      settings: AttributesFormatString=%<OutDataTypeStr>
  single18 : Constant  Value=3.141593  OutDataTypeStr=single
      settings: AttributesFormatString=%<OutDataTypeStr>
  single19 : Constant  Value=360  OutDataTypeStr=single
      settings: AttributesFormatString=%<OutDataTypeStr>
  single2 : Constant  Value=0  OutDataTypeStr=single
      settings: AttributesFormatString=%<OutDataTypeStr>
  single20 : Constant  OutDataTypeStr=single
      settings: AttributesFormatString=%<OutDataTypeStr>
  single21 : Constant  Value=-1  OutDataTypeStr=single
      settings: AttributesFormatString=%<OutDataTypeStr>
  single22 : Constant  Value=0  OutDataTypeStr=single
      settings: AttributesFormatString=%<OutDataTypeStr>
  single3 : Constant  Value=-180  OutDataTypeStr=single
      settings: AttributesFormatString=%<OutDataTypeStr>
  single4 : Constant  Value=-90  OutDataTypeStr=single
      settings: AttributesFormatString=%<OutDataTypeStr>
  single5 : Constant  Value=-270  OutDataTypeStr=single
      settings: AttributesFormatString=%<OutDataTypeStr>
  single7 : Constant  OutDataTypeStr=single
      settings: AttributesFormatString=%<OutDataTypeStr>
  single8 : Constant  Value=-1  OutDataTypeStr=single
      settings: AttributesFormatString=%<OutDataTypeStr>
  single9 : Constant  Value=0  OutDataTypeStr=single
      settings: AttributesFormatString=%<OutDataTypeStr>
  uint1 : Constant  OutDataTypeStr=uint8
      settings: AttributesFormatString=%<OutDataTypeStr>
  uint2 : Constant  Value=4  OutDataTypeStr=uint8
      settings: AttributesFormatString=%<OutDataTypeStr>
  uint3 : Constant  Value=3  OutDataTypeStr=uint8
      settings: AttributesFormatString=%<OutDataTypeStr>
  uint4 : Constant  Value=2  OutDataTypeStr=uint8
      settings: AttributesFormatString=%<OutDataTypeStr>
  uint5 : Constant  OutDataTypeStr=uint8
      settings: AttributesFormatString=%<OutDataTypeStr>
  uint6 : Constant  Value=2  OutDataTypeStr=uint8
      settings: AttributesFormatString=%<OutDataTypeStr>
  uint7 : Constant  Value=3  OutDataTypeStr=uint8
      settings: AttributesFormatString=%<OutDataTypeStr>
  uint8 : Constant  Value=4  OutDataTypeStr=uint8
      settings: AttributesFormatString=%<OutDataTypeStr>
  out : Outport
  wires:
  single22/1 -> Multiport Switch4/6
  Switch6/1 -> Switch5/3
  single3/1 -> GreaterOrEqual5/2
  AbsITK/1 -> Multiport Switch3/3
  Multiport Switch2/1 -> Product2/1
  single5/1 -> GreaterOrEqual4/2
  Switch1/1 -> out/1
  Switch5/1 -> Multiport Switch4/1, Multiport Switch3/1
  Subtract5/1 -> AbsITK/1, Multiport Switch3/4
  single2/1 -> GreaterOrEqual3/2
  Switch7/1 -> Switch6/3
  Switch2/1 -> Multiport Switch2/1, Multiport Switch1/1
  GreaterOrEqual4/1 -> Switch5/2
  Subtract3/1 -> GreaterOrEqual3/1, AbsITK1/1, Subtract5/1, Subtract4/1, GreaterOrEqual6/1, GreaterOrEqual5/1, GreaterOrEqual4/1, Subtract2/2, Subtract1/1, Subtract/2, Multiport Switch1/2, GreaterOrEqual2/1, GreaterOrEqual1/1, GreaterOrEqual/1
  Product4/1 -> Divide/1, Subtract3/1  "deg"
  GreaterOrEqual1/1 -> Switch3/2
  uint5/1 -> Switch4/3
  Subtract1/1 -> Multiport Switch1/4
  Product2/1 -> Switch1/1
  single6/1 -> Subtract/1
  single7/1 -> Multiport Switch2/2, Multiport Switch2/3
  Subtract2/1 -> Multiport Switch1/5
  Product1/1 -> Subtract3/2
  single14/1 -> Subtract1/2
  uint2/1 -> Switch2/1
  single12/1 -> GreaterOrEqual/2
  Switch3/1 -> Switch2/3
  single10/1 -> GreaterOrEqual1/2
  single8/1 -> Multiport Switch2/4, Multiport Switch2/5
  single15/1 -> Subtract2/1
  Multiport Switch3/1 -> 1-D Lookup Table2/1
  Subtract4/1 -> Multiport Switch3/2
  GreaterOrEqual2/1 -> Switch4/2
  GreaterOrEqual5/1 -> Switch6/2
  GreaterOrEqual6/1 -> Switch7/2
  uint7/1 -> Switch7/1
  Multiport Switch1/1 -> 1-D Lookup Table3/1
  uint4/1 -> Switch4/1
  uint8/1 -> Switch7/3
  GreaterOrEqual3/1 -> Switch1/2
  single21/1 -> Multiport Switch4/5, Multiport Switch4/4
  uint1/1 -> Switch5/1
  Divide/1 -> Rounding Function/1
  uint3/1 -> Switch3/1
  Product3/1 -> Switch1/3
  single1/1 -> Product1/2, Divide/2
  AbsITK1/1 -> Multiport Switch3/5
  1-D Lookup Table3/1 -> Product2/2
  Multiport Switch4/1 -> Product3/1
  single19/1 -> Subtract4/2
  single20/1 -> Multiport Switch4/3, Multiport Switch4/2
  Switch4/1 -> Switch3/3
  Rounding Function/1 -> Product1/1
  single9/1 -> Multiport Switch2/6
  1-D Lookup Table2/1 -> Product3/2
  Subtract/1 -> Multiport Switch1/3
  GreaterOrEqual/1 -> Switch2/2
  uint6/1 -> Switch6/1
  single11/1 -> GreaterOrEqual2/2
  single17/1 -> Subtract5/2
  single4/1 -> GreaterOrEqual6/2
  rad/1 -> Divide1/1
  single18/1 -> Divide1/2
  Divide1/1 -> Product4/1
  single23/1 -> Product4/2
